simulink library "Controllers"  (R2016b)
settings: Solver=VariableStepAuto  StartTime=0.0  StopTime=10.0  RelTol=1e-3
undefined symbols (not defined in the file or in its folder): CRM
libraries: lib_Sim_CRM x6, Reinterpolation x2
settings Model: Creator=cava_da  LastModifiedBy=cava_da
settings DataIOCC: ReturnWorkspaceOutputs=on
settings SFSimCC: SimUseLocalCustomCode=on
settings RTWCC: RTWUseLocalCustomCode=on

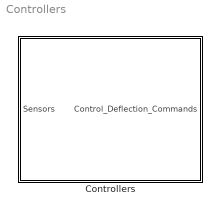
== system Controllers ==
  Controllers : Subsystem

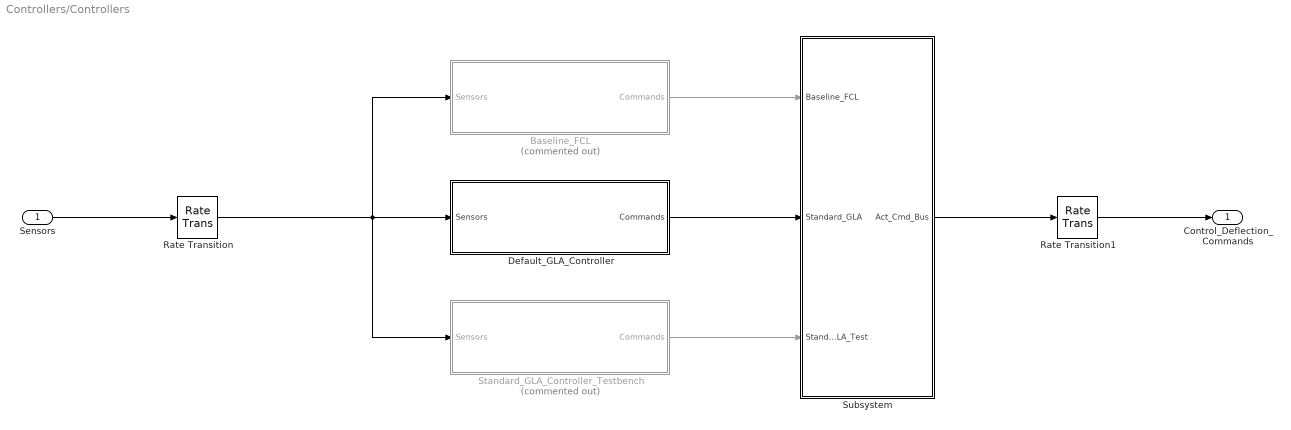
== system Controllers/Controllers ==
  Sensors : Inport
  Baseline_FCL : Subsystem  Commented=on
  Default_GLA_Controller : Subsystem
  Rate Transition : RateTransition  OutPortSampleTime=CRM.FCS.SampleTime
  Rate Transition1 : RateTransition  OutPortSampleTime=SimConfig.SampleTime
  Standard_GLA_Controller_Testbench : Subsystem  Commented=on
  Subsystem : Subsystem
  Control_Deflection_Commands : Outport
  wires:
  Sensors/1 -> Rate Transition/1
  Rate Transition1/1 -> Control_Deflection_Commands/1
  Rate Transition/1 -> Standard_GLA_Controller_Testbench/1(Sensors), Default_GLA_Controller/1(Sensors), Baseline_FCL/1(Sensors)
  Baseline_FCL/1(Commands) -> Subsystem/1(Baseline_FCL)
  Default_GLA_Controller/1(Commands) -> Subsystem/2(Standard_GLA)
  Subsystem/1(Act_Cmd_Bus) -> Rate Transition1/1
  Standard_GLA_Controller_Testbench/1(Commands) -> Subsystem/3(Standard_GLA_Test)

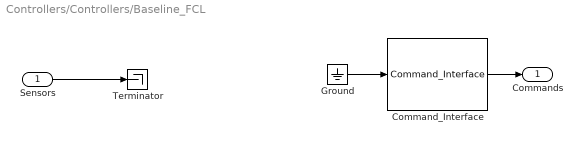
== system Controllers/Controllers/Baseline_FCL ==
  Sensors : Inport
  Command_Interface : lib_Sim_CRM/Command_Interface  SystemSampleTime=-1
  Ground : Ground
  Terminator : Terminator
  Commands : Outport
  wires:
  Sensors/1 -> Terminator/1
  Ground/1 -> Command_Interface/1
  Command_Interface/1 -> Commands/1

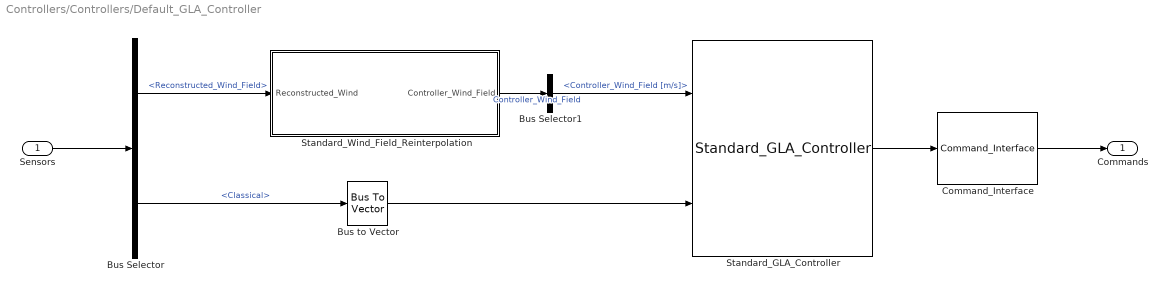
== system Controllers/Controllers/Default_GLA_Controller ==
  Sensors : Inport
  Bus Selector : BusSelector  OutputSignals=Reconstructed_Wind_Field,Classical
  Bus Selector1 : BusSelector  OutputSignals=Controller_Wind_Field [m/s]
  Bus to Vector : BusToVector
  Command_Interface : lib_Sim_CRM/Command_Interface  SystemSampleTime=-1
  Standard_GLA_Controller : lib_Sim_CRM/Standard_GLA_Controller  glaName=CRM.FCS.Controller_Data.CRM_FFGLA_Default
  Standard_Wind_Field_Reinterpolation : Subsystem  mask(Controller Wind Field Reinterpolation){GLA=CRM.FCS.Controller_Data.CRM_FFGLA_Default}
      mask prompts: GLA "Insert GLA Controller structure:"
      mask help: Reinterpolates the estimated wind field to fit the wind field inputs required by a standard GLA controller.
  Commands : Outport
  wires:
  Bus to Vector/1 -> Standard_GLA_Controller/2
  Bus Selector/2 -> Bus to Vector/1  "<Classical>"
  Bus Selector/1 -> Standard_Wind_Field_Reinterpolation/1(Reconstructed_Wind)  "<Reconstructed_Wind_Field>"
  Standard_GLA_Controller/1 -> Command_Interface/1
  Sensors/1 -> Bus Selector/1
  Command_Interface/1 -> Commands/1
  Bus Selector1/1 -> Standard_GLA_Controller/1  "<Controller_Wind_Field [m/s]>"
  Standard_Wind_Field_Reinterpolation/1(Controller_Wind_Field) -> Bus Selector1/1  "Controller_Wind_Field"

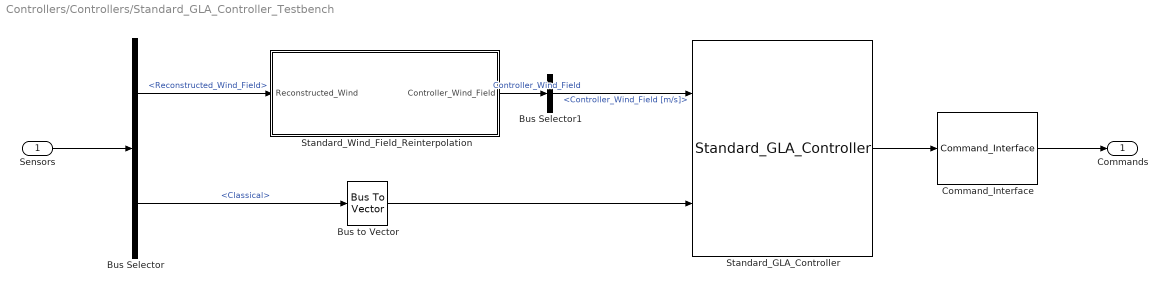
== system Controllers/Controllers/Standard_GLA_Controller_Testbench ==
  Sensors : Inport
  Bus Selector : BusSelector  OutputSignals=Reconstructed_Wind_Field,Classical
  Bus Selector1 : BusSelector  OutputSignals=Controller_Wind_Field [m/s]
  Bus to Vector : BusToVector
  Command_Interface : lib_Sim_CRM/Command_Interface  SystemSampleTime=-1
  Standard_GLA_Controller : lib_Sim_CRM/Standard_GLA_Controller  glaName=CRM.FCS.Controller_Data.CRM_FFGLA_Test
  Standard_Wind_Field_Reinterpolation : Subsystem  mask(Controller Wind Field Reinterpolation){GLA=CRM.FCS.Controller_Data.CRM_FFGLA_Test}
      mask prompts: GLA "Insert GLA Controller structure:"
      mask help: Reinterpolates the estimated wind field to fit the wind field inputs required by a standard GLA controller.
  Commands : Outport
  wires:
  Standard_Wind_Field_Reinterpolation/1(Controller_Wind_Field) -> Bus Selector1/1  "Controller_Wind_Field"
  Bus Selector1/1 -> Standard_GLA_Controller/1  "<Controller_Wind_Field [m/s]>"
  Command_Interface/1 -> Commands/1
  Sensors/1 -> Bus Selector/1
  Standard_GLA_Controller/1 -> Command_Interface/1
  Bus Selector/1 -> Standard_Wind_Field_Reinterpolation/1(Reconstructed_Wind)  "<Reconstructed_Wind_Field>"
  Bus Selector/2 -> Bus to Vector/1  "<Classical>"
  Bus to Vector/1 -> Standard_GLA_Controller/2

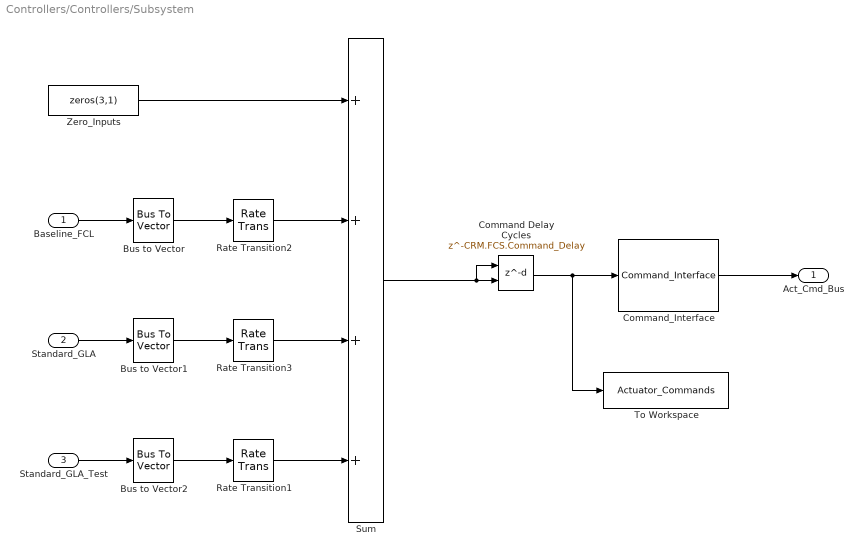
== system Controllers/Controllers/Subsystem ==
  Baseline_FCL : Inport
  Standard_GLA : Inport  Port=2
  Standard_GLA_Test : Inport  Port=3
  Bus to Vector : BusToVector
  Bus to Vector1 : BusToVector
  Bus to Vector2 : BusToVector
  Command Delay Cycles : Delay  DelayLength=CRM.FCS.Command_Delay  InitialConditionSource=Input port
      settings: InputPortMap=u0,p4
  Command_Interface : lib_Sim_CRM/Command_Interface  SystemSampleTime=-1
  Rate Transition1 : RateTransition  OutPortSampleTime=CRM.FCS.SampleTime
  Rate Transition2 : RateTransition  OutPortSampleTime=CRM.FCS.SampleTime
  Rate Transition3 : RateTransition  OutPortSampleTime=CRM.FCS.SampleTime
  Sum : Sum  Inputs=++++
  To Workspace : ToWorkspace  VariableName=Actuator_Commands  SaveFormat=Structure With Time  SampleTime=-1
      settings: Decimation=SimConfig.Logging.DecimationFactor
  Zero_Inputs : Constant  Value=zeros(3,1)
  Act_Cmd_Bus : Outport
  wires:
  Rate Transition3/1 -> Sum/3
  Rate Transition2/1 -> Sum/2
  Standard_GLA/1 -> Bus to Vector1/1
  Sum/1 -> Command Delay Cycles/1, Command Delay Cycles/2
  Baseline_FCL/1 -> Bus to Vector/1
  Command_Interface/1 -> Act_Cmd_Bus/1
  Command Delay Cycles/1 -> To Workspace/1, Command_Interface/1
  Zero_Inputs/1 -> Sum/1
  Bus to Vector/1 -> Rate Transition2/1
  Bus to Vector1/1 -> Rate Transition3/1
  Bus to Vector2/1 -> Rate Transition1/1
  Standard_GLA_Test/1 -> Bus to Vector2/1
  Rate Transition1/1 -> Sum/4

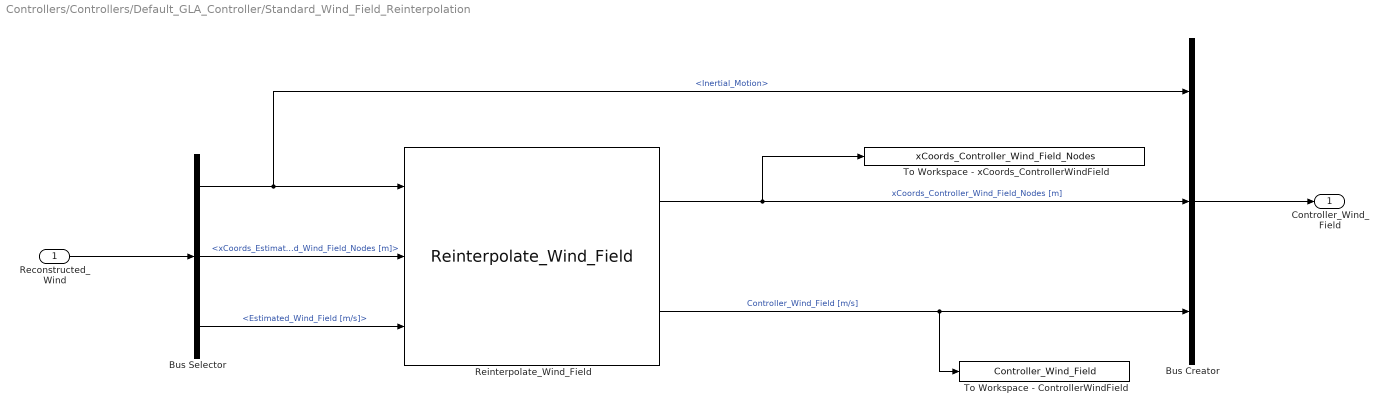
== system Controllers/Controllers/Default_GLA_Controller/Standard_Wind_Field_Reinterpolation ==
  Reconstructed_Wind : Inport
  Bus Creator : BusCreator  Inputs=3
  Bus Selector : BusSelector  OutputSignals=Inertial_Motion,xCoords_Estimated_Wind_Field_Nodes [m],Estimated_Wind_Field [m/s]
  Reinterpolate_Wind_Field : Reinterpolation/Reinterpolate_Wind_Field  t_coords_reinterp=GLA.WindEst.t_coords_ctrl
  To Workspace - ControllerWindField : ToWorkspace  VariableName=Controller_Wind_Field  SaveFormat=Structure With Time  SampleTime=-1
      settings: Decimation=SimConfig.Logging.DecimationFactor
  To Workspace - xCoords_ControllerWindField : ToWorkspace  VariableName=xCoords_Controller_Wind_Field_Nodes  SaveFormat=Structure With Time  SampleTime=-1
      settings: Decimation=SimConfig.Logging.DecimationFactor
  Controller_Wind_Field : Outport
  wires:
  Bus Selector/3 -> Reinterpolate_Wind_Field/3  "<Estimated_Wind_Field [m/s]>"
  Bus Selector/2 -> Reinterpolate_Wind_Field/2  "<xCoords_Estimated_Wind_Field_Nodes [m]>"
  Reconstructed_Wind/1 -> Bus Selector/1
  Reinterpolate_Wind_Field/2 -> To Workspace - ControllerWindField/1, Bus Creator/3  "Controller_Wind_Field [m/s]"
  Bus Selector/1 -> Bus Creator/1, Reinterpolate_Wind_Field/1  "<Inertial_Motion>"
  Bus Creator/1 -> Controller_Wind_Field/1
  Reinterpolate_Wind_Field/1 -> Bus Creator/2, To Workspace - xCoords_ControllerWindField/1  "xCoords_Controller_Wind_Field_Nodes [m]"

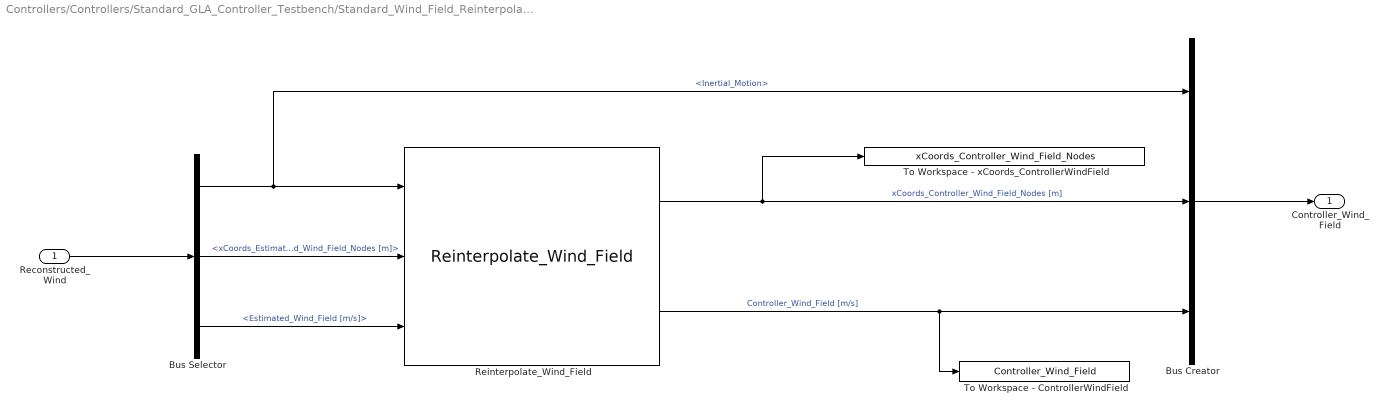
== system Controllers/Controllers/Standard_GLA_Controller_Testbench/Standard_Wind_Field_Reinterpolation ==
  Reconstructed_Wind : Inport
  Bus Creator : BusCreator  Inputs=3
  Bus Selector : BusSelector  OutputSignals=Inertial_Motion,xCoords_Estimated_Wind_Field_Nodes [m],Estimated_Wind_Field [m/s]
  Reinterpolate_Wind_Field : Reinterpolation/Reinterpolate_Wind_Field  t_coords_reinterp=GLA.WindEst.t_coords_ctrl
  To Workspace - ControllerWindField : ToWorkspace  VariableName=Controller_Wind_Field  SaveFormat=Structure With Time  SampleTime=-1
      settings: Decimation=SimConfig.Logging.DecimationFactor
  To Workspace - xCoords_ControllerWindField : ToWorkspace  VariableName=xCoords_Controller_Wind_Field_Nodes  SaveFormat=Structure With Time  SampleTime=-1
      settings: Decimation=SimConfig.Logging.DecimationFactor
  Controller_Wind_Field : Outport
  wires:
  Reinterpolate_Wind_Field/1 -> To Workspace - xCoords_ControllerWindField/1, Bus Creator/2  "xCoords_Controller_Wind_Field_Nodes [m]"
  Bus Creator/1 -> Controller_Wind_Field/1
  Bus Selector/1 -> Reinterpolate_Wind_Field/1, Bus Creator/1  "<Inertial_Motion>"
  Reinterpolate_Wind_Field/2 -> Bus Creator/3, To Workspace - ControllerWindField/1  "Controller_Wind_Field [m/s]"
  Reconstructed_Wind/1 -> Bus Selector/1
  Bus Selector/2 -> Reinterpolate_Wind_Field/2  "<xCoords_Estimated_Wind_Field_Nodes [m]>"
  Bus Selector/3 -> Reinterpolate_Wind_Field/3  "<Estimated_Wind_Field [m/s]>"
